simulink model "Model1_Sarah"  (R2023b)
settings: Solver=FixedStepAuto  StartTime=0.0  StopTime=Inf  FixedStep=1e-4  RelTol=1e-3
PostLoadFcn:
  | if any(exist('dsrtsu_mdlpostloadfcn', 'file') ~= 0), dsrtsu_mdlpostloadfcn('Execute', bdroot); end
InitFcn:
  | , if any(exist('rtifpga_mdlclblib', 'file') ~= 0), rtifpga_mdlclblib('Init', bdroot); end,
  | , if any(exist('dsmpb_private', 'file') ~= 0), dsmpb_private('dsmpb_mdlclblib', 'Init', bdroot); end,
  | load('LUT_BRUSA_jax_grad.mat')
  | load('daten_nichtlinear_interpoliert.mat')
  | load('Maschinendaten.mat')
  | load('PI_Controller.mat')
  | load('Nonlinear_IPMSM.mat')
values from neighbouring files (symbols this model uses):
  I_max = 170    [Maschinendaten.mat]    (also in Maschinendaten_Vorgabe.m; test_ModelParameters.m = evalin('base', 'I_max'); test_StrategySelection.m = tc.readConstant(tc.BLK_Imax))
  ID = [-250 -250 -250 -250 -250 -250 -250 -250 -250 -250 -250 -250 ... (10000 elements, 100x100)]    [daten_nichtlinear_interpoliert.mat]
  id_fine = linspace(min(id_vec), max(id_vec), 100)    [Messdaten_Interpoliert.m]    (also in daten_nichtlinear_interpoliert.mat = [-250 -247.474747475 -244.949494949 -242.424242424 -239.8989)
  IQ = [-250 -244.949494949 -239.898989899 -234.848484848 -229.797979798 -224.747474747 -219.696969697 -214.646464646 -209.595959596 -204.545454545 -199.494949495 -194.444444444 ... (10000 elements, 100x100)]    [daten_nichtlinear_interpoliert.mat]
  iq_fine = linspace(min(iq_vec), max(iq_vec), 100)    [Messdaten_Interpoliert.m]    (also in daten_nichtlinear_interpoliert.mat = [-250 -244.949494949 -239.898989899 -234.848484848 -229.7979)
  Ld = Ldd_fine    [Messdaten_Interpoliert.m]    (also in daten_nichtlinear_interpoliert.mat = [0.000225276031415 0.000225750625371 0.000226241749969 0.000)
  Lm = Lm_fine1    [Messdaten_Interpoliert.m]    (also in daten_nichtlinear_interpoliert.mat = [1.34827571578e-05 1.31035668506e-05 1.23153687442e-05 1.146)
  Lq = Lqq_fine    [Messdaten_Interpoliert.m]    (also in daten_nichtlinear_interpoliert.mat = [0.000286039721686 0.000286453471045 0.000286025480511 0.000)
  n_max = 11000    [Maschinendaten.mat]    (also in Maschinendaten_Vorgabe.m; test_ModelParameters.m = evalin('base', 'n_max'); test_StrategySelection.m = tc.readConstant(tc.BLK_nmax))
  p = 3    [Maschinendaten.mat]    (also in Maschinendaten_Vorgabe.m; Messdaten_Interpoliert.m; test_ModelParameters.m = evalin('base', 'p'))
  PSID = Psid_fine    [Messdaten_Interpoliert.m]    (also in daten_nichtlinear_interpoliert.mat = [0.00602681114795 0.00609490588107 0.00615917040906 0.006219)
  PSIQ = PSIQ1 - PSIQ1(iq0_idx,:)    [Messdaten_Interpoliert.m]    (also in daten_nichtlinear_interpoliert.mat = [-0.151946994742 -0.150499709177 -0.149057806808 -0.14762041)
  Rs = 0.018    [Maschinendaten.mat]    (also in Maschinendaten_Vorgabe.m; test_ModelParameters.m = evalin('base', 'Rs'))
  U_dc = 560    [Maschinendaten.mat]    (also in Maschinendaten_Vorgabe.m; test_ModelParameters.m = evalin('base', 'U_dc'))
  U_max = 323.316150746    [Maschinendaten.mat]    (also in Maschinendaten_Vorgabe.m = U_dc / sqrt(3); test_ModelParameters.m = evalin('base', 'U_max'))
libraries: dsmpblib x6
(part 1 of 2)
PreSaveFcn:
  | , if any(exist('dsmpb_private', 'file') ~= 0), dsmpb_private('dsmpb_mdlclblib', 'PreSave', bdroot); end,
CloseFcn:
  | , if any(exist('dsmpb_private', 'file') ~= 0), dsmpb_private('dsmpb_mdlclblib', 'Close', bdroot); end,
settings Model: DSRTSU_INTERNAL_RTIFPGA=210  DSRTSU_INTERNAL_RTISTBM_VER=24.2  DSMPB_ID_DATA={'227',struct('BlockId','b1d00881-2476-43fd-8fde-9f6f39539870396','SignalIds',{{'b1d00881-2476-43fd-8fde-9f6f39539870396_1'}}),'228',struct('BlockId','b1d00881-2476-43fd-8fde-9f6f39539870397','SignalIds',{{'b1d00881-2476-43fd-8fde-9f6f39539870397_1'}}),'229',struct('BlockId','b1d00881-2476-43fd-8fde-9f6f39539870398','SignalIds',{{'b1d00881-2476-43fd-8fde-9f6f39539870398_1'}}),'230',struct('BlockId','b1d00881-2476-43fd-8fde-9f6f39539870399','SignalIds',{{'b1d00881-2476-43fd-8fde-9f6f39539870399_1'}}),'231',struct('BlockId','b1d00881-2476-43fd-8fde-9f6f39539870400','SignalIds',{{'b1d00881-2476-43fd-8fde-9f6f39539870400_1'}}),'232',struct('BlockId','b1d00881-2476-43fd-8fde-9f6f39539870401','SignalIds',{{'b1d00881-2476-43fd-8fde-9f6f39539870401_1'}})}  Creator=Student  LastModifiedBy=Student
settings OptimizationCC: BlockReduction=off  ConditionallyExecuteInputs=off  OptimizeBlockIOStorage=off  BufferReuse=off
settings DebuggingCC: TasksWithSamePriorityMsg=none
settings HardwareCC: ProdBitPerLong=64  ProdLargestAtomicInteger=Integer  ProdWordSize=32  ProdLongLongMode=on  ProdHWDeviceType=Custom Processor->Custom
settings ModelReferenceCC: EnableParallelModelReferenceBuilds=on
settings RTWCC: Description=dSPACE Target DSRT - Generates SIC files for import by ConfigurationDesk and VEOS. Provides code generation for Simulink models imported in ConfigurationDesk.  SystemTargetFile=dsrt.tlc  GenCodeOnly=on  MakeCommand=make_dsrt  TemplateMakefile=dsrt_default_tmf  RTWVerbose=off
settings STFCustomTargetCC: ParMdlRefBuildCompliant=on  SystemTargetFile=dsrt.tlc
settings GRTTargetCC: CompOptLevelCompliant=off  ConcurrentExecutionCompliant=off  CombineOutputUpdateFcns=off  MatFileLogging=off  CPPClassGenCompliant=off  UseToolchainInfoCompliant=off

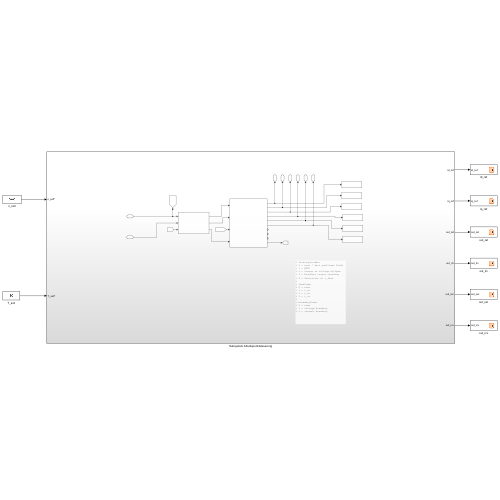
[thumbnail: Simulink's stored preview of the top-level diagram]
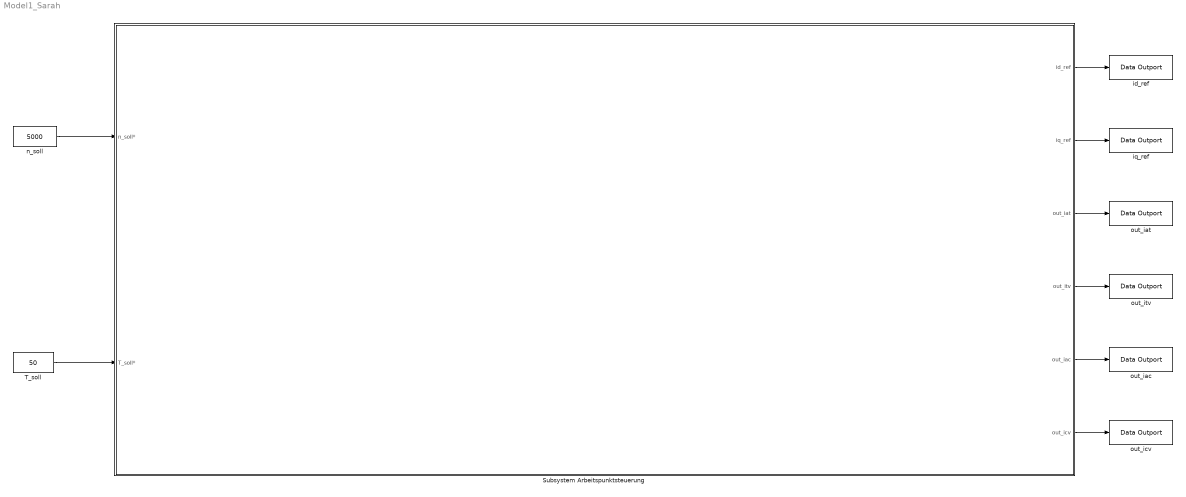
== system Model1_Sarah ==
  Subsystem Arbeitspunktsteuerung : Subsystem
  T_soll : Constant  Value=50
  id_ref : dsmpblib/Data Outport  Priority=-10000
      settings: SourceProductName=dSPACE Model Interface Package for Simulink (MIPS)
  iq_ref : dsmpblib/Data Outport  Priority=-10000
      settings: SourceProductName=dSPACE Model Interface Package for Simulink (MIPS)
  n_soll : Constant  Value=5000
  out_iac : dsmpblib/Data Outport  Priority=-10000
      settings: SourceProductName=dSPACE Model Interface Package for Simulink (MIPS)
  out_iat : dsmpblib/Data Outport  Priority=-10000
      settings: SourceProductName=dSPACE Model Interface Package for Simulink (MIPS)
  out_icv : dsmpblib/Data Outport  Priority=-10000
      settings: SourceProductName=dSPACE Model Interface Package for Simulink (MIPS)
  out_itv : dsmpblib/Data Outport  Priority=-10000
      settings: SourceProductName=dSPACE Model Interface Package for Simulink (MIPS)
  wires:
  Subsystem Arbeitspunktsteuerung/3(out_iat) -> out_iat/1
  Subsystem Arbeitspunktsteuerung/4(out_itv) -> out_itv/1
  Subsystem Arbeitspunktsteuerung/5(out_iac) -> out_iac/1
  Subsystem Arbeitspunktsteuerung/6(out_icv) -> out_icv/1
  n_soll/1 -> Subsystem Arbeitspunktsteuerung/1(n_soll*)
  T_soll/1 -> Subsystem Arbeitspunktsteuerung/2(T_soll*)
  Subsystem Arbeitspunktsteuerung/1(id_ref) -> id_ref/1
  Subsystem Arbeitspunktsteuerung/2(iq_ref) -> iq_ref/1

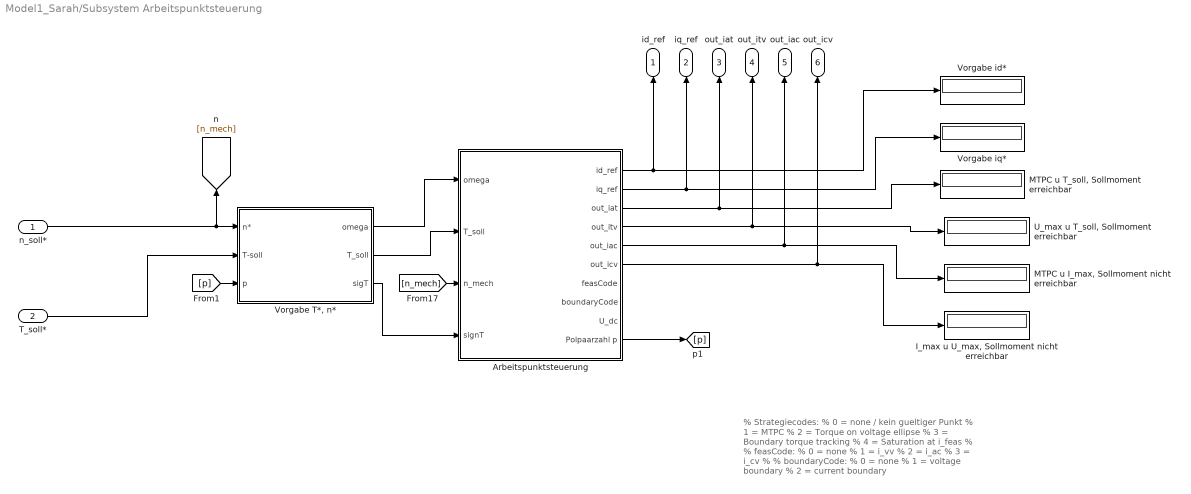
== system Model1_Sarah/Subsystem Arbeitspunktsteuerung ==
  note: % Strategiecodes:
      | % 0 = none / kein gueltiger Punkt
      | % 1 = MTPC
      | % 2 = Torque on voltage ellipse
      | % 3 = Boundary torque tracking
      | % 4 = Saturation at i_feas
      | %
      | % feasCode:
      | % 0 = none
      | % 1 = i_vv
      | % 2 = i_ac
      | % 3 = i_cv
      | %
      | % boundaryCode:
      | % 0 = none
      | % 1 = voltage boundary
      | % 2 = current boundary
  n_soll* : Inport
  T_soll* : Inport  Port=2
  Arbeitspunktsteuerung : Subsystem
  "I_max u U_max, Sollmoment nicht erreichbar" : Display
  "MTPC u I_max, Sollmoment nicht erreichbar" : Display
  "MTPC u T_soll, Sollmoment erreichbar" : Display
  "U_max u T_soll, Sollmoment erreichbar" : Display
  "Vorgabe T*, n*" : Subsystem
  Vorgabe id* : Display
  Vorgabe iq* : Display
  id_ref : Outport
  iq_ref : Outport  Port=2
  out_iat : Outport  Port=3
  out_itv : Outport  Port=4
  out_iac : Outport  Port=5
  out_icv : Outport  Port=6
  wires:
  Arbeitspunktsteuerung/10(Polpaarzahl p) -> [p]
  "Vorgabe T*, n*"/1(omega) -> Arbeitspunktsteuerung/1(omega)
  Arbeitspunktsteuerung/5(out_iac) -> "MTPC u I_max, Sollmoment nicht erreichbar"/1, out_iac/1
  "Vorgabe T*, n*"/3(sigT) -> Arbeitspunktsteuerung/4(signT)
  [n_mech] -> Arbeitspunktsteuerung/3(n_mech)
  Arbeitspunktsteuerung/2(iq_ref) -> Vorgabe iq*/1, iq_ref/1
  Arbeitspunktsteuerung/3(out_iat) -> "MTPC u T_soll, Sollmoment erreichbar"/1, out_iat/1
  Arbeitspunktsteuerung/1(id_ref) -> Vorgabe id*/1, id_ref/1
  Arbeitspunktsteuerung/4(out_itv) -> "U_max u T_soll, Sollmoment erreichbar"/1, out_itv/1
  T_soll*/1 -> "Vorgabe T*, n*"/2(T-soll)
  [p] -> "Vorgabe T*, n*"/3(p)
  "Vorgabe T*, n*"/2(T_soll) -> Arbeitspunktsteuerung/2(T_soll)
  n_soll*/1 -> "Vorgabe T*, n*"/1(n*), [n_mech]
  Arbeitspunktsteuerung/6(out_icv) -> "I_max u U_max, Sollmoment nicht erreichbar"/1, out_icv/1

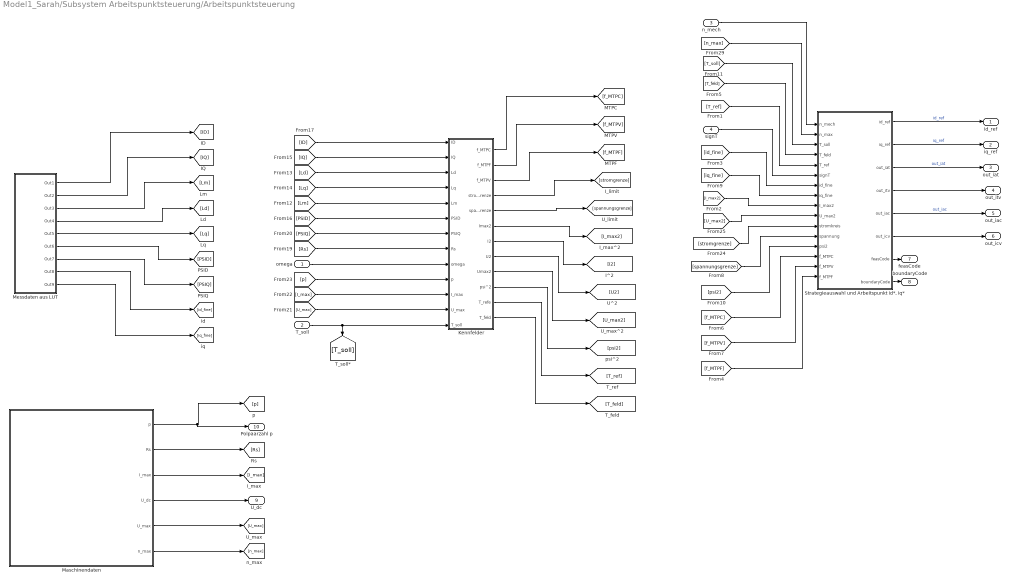
== system Model1_Sarah/Subsystem Arbeitspunktsteuerung/Arbeitspunktsteuerung ==
  omega : Inport
  T_soll : Inport  Port=2
  n_mech : Inport  Port=3
  signT : Inport  Port=4
  Kennfelder : Subsystem  Tag=<DSModel=3_'Model_Sarah'>
      settings: AttributesFormatString=<DSModel='Model_Sarah'>
  Maschinendaten : Subsystem  Tag=<DSModel=5_'Model_Sarah'>
      settings: AttributesFormatString=<DSModel='Model_Sarah'>
  Messdaten aus LUT : Subsystem  Tag=<DSModel=4_'Model_Sarah'>
      settings: AttributesFormatString=<DSModel='Model_Sarah'>
  "Strategieauswahl und Arbeitspunkt id*, iq*" : MATLAB Function  Tag=<DSModel=1_'Model_Sarah'>  TreatAsAtomicUnit=on
      settings: AttributesFormatString=<DSModel='Model_Sarah'>
  id_ref : Outport
  iq_ref : Outport  Port=2
  out_iat : Outport  Port=3
  out_itv : Outport  Port=4
  out_iac : Outport  Port=5
  out_icv : Outport  Port=6
  feasCode : Outport  Port=7
  boundaryCode : Outport  Port=8
  " U_dc" : Outport  Port=9
  Polpaarzahl p : Outport  Port=10
  wires:
  [T_soll] -> "Strategieauswahl und Arbeitspunkt id*, iq*"/3(T_soll)
  "Strategieauswahl und Arbeitspunkt id*, iq*"/7(feasCode) -> feasCode/1
  Kennfelder/9(Umax2) -> [U_max2]
  [stromgrenze] -> "Strategieauswahl und Arbeitspunkt id*, iq*"/11(stromkreis)
  Kennfelder/2(f_MTPF) -> [f_MTPV]
  Messdaten aus LUT/6(Out6) -> [PSID]
  [U_max] -> Kennfelder/12(U_max)
  "Strategieauswahl und Arbeitspunkt id*, iq*"/6(out_icv) -> out_icv/1
  [spannungsgrenze] -> "Strategieauswahl und Arbeitspunkt id*, iq*"/12(spannung)
  Messdaten aus LUT/7(Out7) -> [PSIQ]
  [id_fine] -> "Strategieauswahl und Arbeitspunkt id*, iq*"/7(id_fine)
  Messdaten aus LUT/1(Out1) -> [ID]
  "Strategieauswahl und Arbeitspunkt id*, iq*"/3(out_iat) -> out_iat/1  "out_iat"
  [f_MTPF] -> "Strategieauswahl und Arbeitspunkt id*, iq*"/16(f_MTPF)
  Kennfelder/6(Imax2) -> [I_max2]
  [I_max2] -> "Strategieauswahl und Arbeitspunkt id*, iq*"/9(I_max2)
  signT/1 -> "Strategieauswahl und Arbeitspunkt id*, iq*"/6(signT)
  Messdaten aus LUT/9(Out9) -> [iq_fine]
  "Strategieauswahl und Arbeitspunkt id*, iq*"/5(out_iac) -> out_iac/1  "out_iac"
  omega/1 -> Kennfelder/9(omega)
  Messdaten aus LUT/2(Out2) -> [IQ]
  Maschinendaten/5(U_max) -> [U_max]
  [iq_fine] -> "Strategieauswahl und Arbeitspunkt id*, iq*"/8(iq_fine)
  Kennfelder/8(U2) -> [U2]
  [Lq] -> Kennfelder/4(Lq)
  Kennfelder/3(f_MTPV) -> [f_MTPF]
  [p] -> Kennfelder/10(p)
  Kennfelder/1(f_MTPC) -> [f_MTPC]
  [T_ref] -> "Strategieauswahl und Arbeitspunkt id*, iq*"/5(T_ref)
  "Strategieauswahl und Arbeitspunkt id*, iq*"/2(iq_ref) -> iq_ref/1  "iq_ref"
  Kennfelder/4(stromgrenze) -> [stromgrenze]
  Messdaten aus LUT/8(Out8) -> [id_fine]
  [ID] -> Kennfelder/1(ID)
  Messdaten aus LUT/4(Out4) -> [Ld]
  Kennfelder/12(T_feld) -> [T_feld]
  [psi2] -> "Strategieauswahl und Arbeitspunkt id*, iq*"/13(psi2)
  "Strategieauswahl und Arbeitspunkt id*, iq*"/8(boundaryCode) -> boundaryCode/1
  [PSIQ] -> Kennfelder/7(PSIQ)
  Maschinendaten/1(" p") -> [p], Polpaarzahl p/1
  Maschinendaten/3(" I_max") -> [I_max]
  "Strategieauswahl und Arbeitspunkt id*, iq*"/1(id_ref) -> id_ref/1  "id_ref"
  [f_MTPV] -> "Strategieauswahl und Arbeitspunkt id*, iq*"/15(f_MTPV)
  Kennfelder/5(spannungsgrenze) -> [spannungsgrenze]
  [PSID] -> Kennfelder/6(PSID)
  T_soll/1 -> [T_soll], Kennfelder/13(T_soll)
  [n_max] -> "Strategieauswahl und Arbeitspunkt id*, iq*"/2(n_max)
  Messdaten aus LUT/3(Out3) -> [Lm]
  Kennfelder/11(T_refe) -> [T_ref]
  Messdaten aus LUT/5(Out5) -> [Lq]
  Kennfelder/10(psi^2) -> [psi2]
  [IQ] -> Kennfelder/2(IQ)
  n_mech/1 -> "Strategieauswahl und Arbeitspunkt id*, iq*"/1(n_mech)
  [f_MTPC] -> "Strategieauswahl und Arbeitspunkt id*, iq*"/14(f_MTPC)
  Maschinendaten/6(n_max) -> [n_max]
  [I_max] -> Kennfelder/11(I_max)
  [Lm] -> Kennfelder/5(Lm)
  [T_feld] -> "Strategieauswahl und Arbeitspunkt id*, iq*"/4(T_feld)
  Kennfelder/7(I2) -> [I2]
  Maschinendaten/2(" Rs") -> [Rs]
  Maschinendaten/4(" U_dc") -> " U_dc"/1
  "Strategieauswahl und Arbeitspunkt id*, iq*"/4(out_itv) -> out_itv/1
  [Rs] -> Kennfelder/8(Rs)
  [Ld] -> Kennfelder/3(Ld)
  [U_max2] -> "Strategieauswahl und Arbeitspunkt id*, iq*"/10(U_max2)

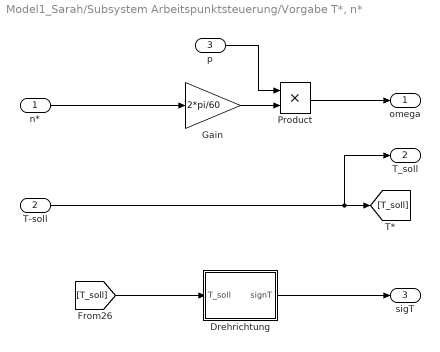
== system Model1_Sarah/Subsystem Arbeitspunktsteuerung/Vorgabe T*, n* ==
  n* : Inport
  T-soll : Inport  Port=2
  p : Inport  Port=3
  Drehrichtung : MATLAB Function  Tag=<DSModel=2_'Model_Sarah'>  TreatAsAtomicUnit=on
      settings: AttributesFormatString=<DSModel='Model_Sarah'>
  Gain : Gain  Gain=2*pi/60
  Product : Product
  omega : Outport
  T_soll : Outport  Port=2
  sigT : Outport  Port=3
  wires:
  p/1 -> Product/1
  Drehrichtung/1(signT) -> sigT/1
  Gain/1 -> Product/2
  n*/1 -> Gain/1
  T-soll/1 -> [T_soll], T_soll/1
  Product/1 -> omega/1
  [T_soll] -> Drehrichtung/1(T_soll)

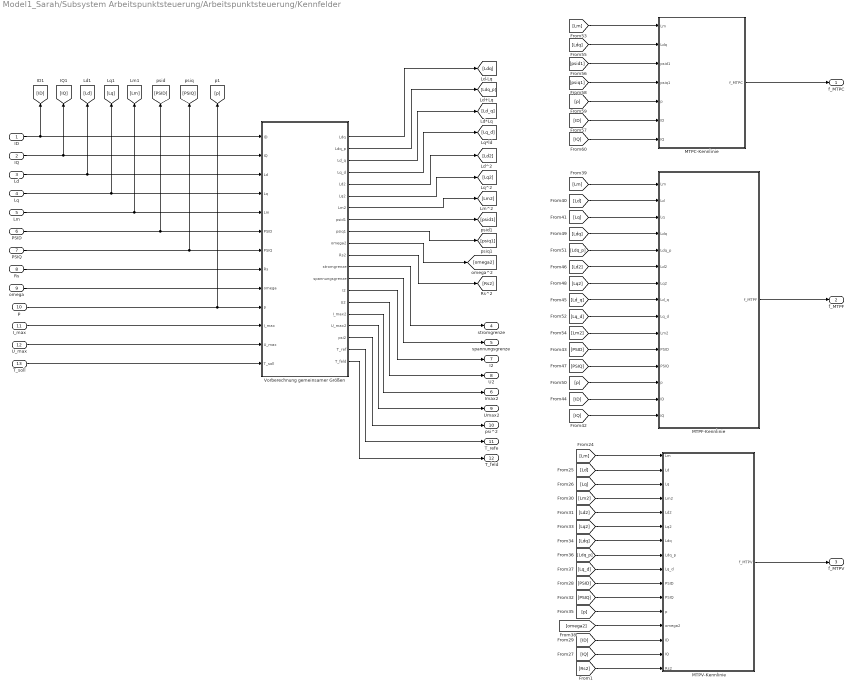
== system Model1_Sarah/Subsystem Arbeitspunktsteuerung/Arbeitspunktsteuerung/Kennfelder ==
  ID : Inport
  IQ : Inport  Port=2
  Ld : Inport  Port=3
  Lq : Inport  Port=4
  Lm : Inport  Port=5
  PSID : Inport  Port=6
  PSIQ : Inport  Port=7
  Rs : Inport  Port=8
  omega : Inport  Port=9
  p : Inport  Port=10
  I_max : Inport  Port=11
  U_max : Inport  Port=12
  T_soll : Inport  Port=13
  " Vorberechnung gemeinsamer Größen" : MATLAB Function  TreatAsAtomicUnit=on
  MTPC-Kennlinie : MATLAB Function  TreatAsAtomicUnit=on
  MTPF-Kennlinie : MATLAB Function  TreatAsAtomicUnit=on
  MTPV-Kennlinie : MATLAB Function  TreatAsAtomicUnit=on
  f_MTPC : Outport
  f_MTPF : Outport  Port=2
  f_MTPV : Outport  Port=3
  stromgrenze : Outport  Port=4
  spannungsgrenze : Outport  Port=5
  Imax2 : Outport  Port=6
  I2 : Outport  Port=7
  U2 : Outport  Port=8
  Umax2 : Outport  Port=9
  psi^2 : Outport  Port=10
  T_refe : Outport  Port=11
  T_feld : Outport  Port=12
  wires:
  T_soll/1 -> " Vorberechnung gemeinsamer Größen"/13(T_soll)
  " Vorberechnung gemeinsamer Größen"/20(T_feld) -> T_feld/1
  " Vorberechnung gemeinsamer Größen"/19(T_ref) -> T_refe/1
  " Vorberechnung gemeinsamer Größen"/18(psi2) -> psi^2/1
  " Vorberechnung gemeinsamer Größen"/16(I_max2) -> Imax2/1
  " Vorberechnung gemeinsamer Größen"/14(I2) -> I2/1
  " Vorberechnung gemeinsamer Größen"/17(U_max2) -> Umax2/1
  " Vorberechnung gemeinsamer Größen"/15(U2) -> U2/1
  [Rs2] -> MTPV-Kennlinie/16(Rs2)
  MTPV-Kennlinie/1(f_MTPV) -> f_MTPV/1
  MTPC-Kennlinie/1(f_MTPC) -> f_MTPC/1
  MTPF-Kennlinie/1(f_MTPF) -> f_MTPF/1
  PSID/1 -> " Vorberechnung gemeinsamer Größen"/6(PSID), [PSID]
  Lm/1 -> " Vorberechnung gemeinsamer Größen"/5(Lm), [Lm]
  U_max/1 -> " Vorberechnung gemeinsamer Größen"/12(U_max)
  Lq/1 -> " Vorberechnung gemeinsamer Größen"/4(Lq), [Lq]
  I_max/1 -> " Vorberechnung gemeinsamer Größen"/11(I_max)
  IQ/1 -> " Vorberechnung gemeinsamer Größen"/2(IQ), [IQ]
  p/1 -> " Vorberechnung gemeinsamer Größen"/10(p), [p]
  PSIQ/1 -> " Vorberechnung gemeinsamer Größen"/7(PSIQ), [PSIQ]
  [Ldq] -> MTPF-Kennlinie/4(Ldq)
  [omega2] -> MTPV-Kennlinie/13(omega2)
  omega/1 -> " Vorberechnung gemeinsamer Größen"/9(omega)
  [Ld2] -> MTPF-Kennlinie/6(Ld2)
  [Lq] -> MTPV-Kennlinie/3(Lq)
  [Lm] -> MTPV-Kennlinie/1(Lm)
  " Vorberechnung gemeinsamer Größen"/7(Lm2) -> [Lm2]
  [Ld] -> MTPF-Kennlinie/2(Ld)
  [Ldq_p] -> MTPV-Kennlinie/8(Ldq_p)
  [Ldq] -> MTPV-Kennlinie/7(Ldq)
  " Vorberechnung gemeinsamer Größen"/3(Ld_q) -> [Ld_q]
  [Lq2] -> MTPV-Kennlinie/6(Lq2)
  [ID] -> MTPV-Kennlinie/14(ID)
  [PSIQ] -> MTPF-Kennlinie/12(PSIQ)
  " Vorberechnung gemeinsamer Größen"/4(Lq_d) -> [Lq_d]
  [p] -> MTPC-Kennlinie/5(p)
  " Vorberechnung gemeinsamer Größen"/8(psid1) -> [psid1]
  [Lq_d] -> MTPV-Kennlinie/9(Lq_d)
  Ld/1 -> " Vorberechnung gemeinsamer Größen"/3(Ld), [Ld]
  [ID] -> MTPF-Kennlinie/14(ID)
  Rs/1 -> " Vorberechnung gemeinsamer Größen"/8(Rs)
  " Vorberechnung gemeinsamer Größen"/1(Ldq) -> [Ldq]
  [Ldq_p] -> MTPF-Kennlinie/5(Ldq_p)
  [IQ] -> MTPV-Kennlinie/15(IQ)
  [PSID] -> MTPV-Kennlinie/10(PSID)
  " Vorberechnung gemeinsamer Größen"/10(omega2) -> [omega2]
  " Vorberechnung gemeinsamer Größen"/13(spannungsgrenze) -> spannungsgrenze/1
  [Lm] -> MTPC-Kennlinie/1(Lm)
  [psiq1] -> MTPC-Kennlinie/4(psiq1)
  [psid1] -> MTPC-Kennlinie/3(psid1)
  [p] -> MTPF-Kennlinie/13(p)
  ID/1 -> " Vorberechnung gemeinsamer Größen"/1(ID), [ID]
  [IQ] -> MTPC-Kennlinie/7(IQ)
  [ID] -> MTPC-Kennlinie/6(ID)
  [IQ] -> MTPF-Kennlinie/15(IQ)
  [Lq2] -> MTPF-Kennlinie/7(Lq2)
  " Vorberechnung gemeinsamer Größen"/12(stromgrenze) -> stromgrenze/1
  " Vorberechnung gemeinsamer Größen"/5(Ld2) -> [Ld2]
  [Ld_q] -> MTPF-Kennlinie/8(Ld_q)
  [Lm] -> MTPF-Kennlinie/1(Lm)
  [PSID] -> MTPF-Kennlinie/11(PSID)
  " Vorberechnung gemeinsamer Größen"/11(Rs2) -> [Rs2]
  [Ld] -> MTPV-Kennlinie/2(Ld)
  " Vorberechnung gemeinsamer Größen"/6(Lq2) -> [Lq2]
  [Lq] -> MTPF-Kennlinie/3(Lq)
  [Lm2] -> MTPF-Kennlinie/10(Lm2)
  [Lq_d] -> MTPF-Kennlinie/9(Lq_d)
  [Ld2] -> MTPV-Kennlinie/5(Ld2)
  [p] -> MTPV-Kennlinie/12(p)
  " Vorberechnung gemeinsamer Größen"/9(psiq1) -> [psiq1]
  [Lm2] -> MTPV-Kennlinie/4(Lm2)
  [PSIQ] -> MTPV-Kennlinie/11(PSIQ)
  " Vorberechnung gemeinsamer Größen"/2(Ldq_p) -> [Ldq_p]
  [Ldq] -> MTPC-Kennlinie/2(Ldq)

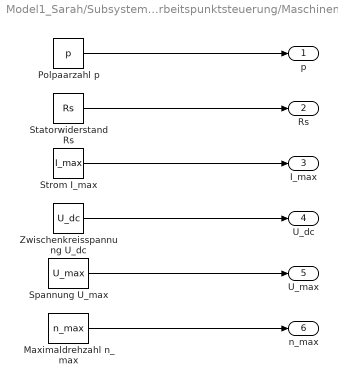
== system Model1_Sarah/Subsystem Arbeitspunktsteuerung/Arbeitspunktsteuerung/Maschinendaten ==
  Maximaldrehzahl n_max : Constant  Value=n_max
  Polpaarzahl p : Constant  Value=p
  Spannung U_max : Constant  Value=U_max
  Statorwiderstand Rs : Constant  Value=Rs
  Strom I_max : Constant  Value=I_max
  Zwischenkreisspannung U_dc : Constant  Value=U_dc
  " p" : Outport
  " Rs" : Outport  Port=2
  " I_max" : Outport  Port=3
  " U_dc" : Outport  Port=4
  U_max : Outport  Port=5
  n_max : Outport  Port=6
  wires:
  Maximaldrehzahl n_max/1 -> n_max/1
  Spannung U_max/1 -> U_max/1
  Statorwiderstand Rs/1 -> " Rs"/1
  Polpaarzahl p/1 -> " p"/1
  Strom I_max/1 -> " I_max"/1
  Zwischenkreisspannung U_dc/1 -> " U_dc"/1

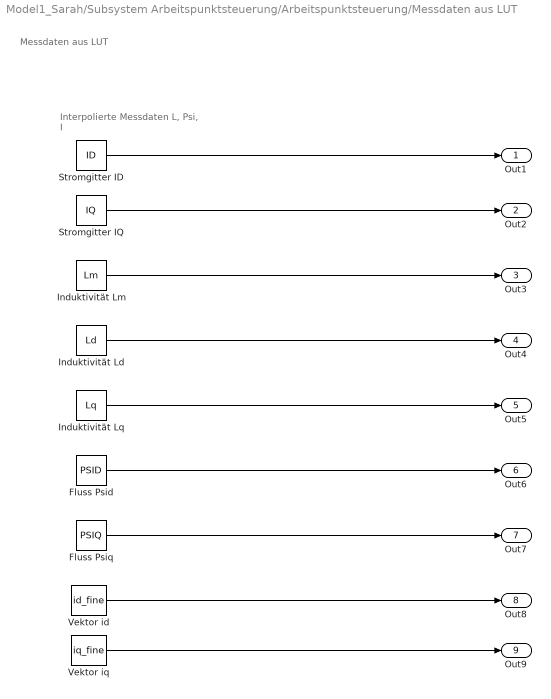
== system Model1_Sarah/Subsystem Arbeitspunktsteuerung/Arbeitspunktsteuerung/Messdaten aus LUT ==
  note: Messdaten aus LUT
  note: Interpolierte Messdaten L, Psi, I
  Fluss Psid : Constant  Value=PSID
  Fluss Psiq : Constant  Value=PSIQ
  Induktivität Ld : Constant  Value=Ld
  Induktivität Lm : Constant  Value=Lm
  Induktivität Lq : Constant  Value=Lq
  Stromgitter ID : Constant  Value=ID
  Stromgitter IQ : Constant  Value=IQ
  Vektor id : Constant  Value=id_fine
  Vektor iq : Constant  Value=iq_fine
  Out1 : Outport
  Out2 : Outport  Port=2
  Out3 : Outport  Port=3
  Out4 : Outport  Port=4
  Out5 : Outport  Port=5
  Out6 : Outport  Port=6
  Out7 : Outport  Port=7
  Out8 : Outport  Port=8
  Out9 : Outport  Port=9
  wires:
  Vektor id/1 -> Out8/1
  Vektor iq/1 -> Out9/1
  Stromgitter ID/1 -> Out1/1
  Stromgitter IQ/1 -> Out2/1
  Fluss Psid/1 -> Out6/1
  Fluss Psiq/1 -> Out7/1
  Induktivität Lm/1 -> Out3/1
  Induktivität Ld/1 -> Out4/1
  Induktivität Lq/1 -> Out5/1

== matlab function Model1_Sarah/Subsystem Arbeitspunktsteuerung/Arbeitspunktsteuerung/Strategieauswahl und Arbeitspunkt id*, iq* ==
  data: n_mech input; n_max input; T_soll input; T_feld input; T_ref input; signT input; id_fine input; iq_fine input; I_max2 input; U_max2 input; stromkreis input; spannung input; psi2 input; f_MTPC input; f_MTPV input; f_MTPF input; id_ref output; iq_ref output; out_iat output; out_itv output; out_iac output; out_icv output; feasCode output; boundaryCode output
%% Strategieauswahl gemäß Flowchart und Bestimmung Arbeitspunkt id*, iq*
% Interpolation, Charak. Punkte, Flowchart-Logik, Nachverfeinerung

%% FUNKTIONIERT NICHT KORREKT STAND 25.06.2026
% Bei T*= 70, n*=10000 wird nicht itv gewählt

function [id_ref, iq_ref, out_iat, out_itv, out_iac, out_icv, feasCode, boundaryCode] = fcn( ...
     n_mech, n_max, T_soll, T_feld, T_ref, signT,...
     id_fine, iq_fine, I_max2, U_max2, ...
     stromkreis,spannung, psi2, f_MTPC, f_MTPV, f_MTPF)

% Strategiecodes, da keine Textausgabe möglich:
% Fälle:
%   out_iat = 1  -> MTPC ∩ T_soll, Sollmoment erreichbar
%   out_itv = 1  -> U_max ∩ T_soll, Sollmoment erreichbar
%   out_iac = 1  -> MTPC ∩ I_max, Sollmoment nicht erreichbar
%   out_icv = 1  -> I_max ∩ U_max, Sollmoment nicht erreichbar
%
% feasCode:
% 0 = none
% 1 = i_vv
% 2 = i_ac
% 3 = i_cv
%
% boundaryCode:
% 0 = none
% 1 = voltage boundary
% 2 = current boundary

%% Konstanten fuer Root-/Mode-Codes
ROOT_AC = 1;
ROOT_VV = 2;
ROOT_AV = 3;
ROOT_CV = 4;
ROOT_AT = 5;
ROOT_TV = 6;

MODE_INTERIOR = 1;
MODE_BOUNDARY = 2;
MODE_VOLTAGE  = 3;

BND_NONE    = 0;
BND_VOLTAGE = 1;
BND_CURRENT = 2;

%% Initialisierung
id_ref = 0.0;
iq_ref = 0.0;
feasCode = int32(0);
boundaryCode = int32(0);

i_ref  = [NaN NaN];
i_feas = [NaN NaN];

out_iat = 0.0;
out_itv = 0.0;
out_iac = 0.0;
out_icv = 0.0;

%% Schutz
if n_mech > n_max
    id_ref = 0.0;
    iq_ref = 0.0;
    feasCode = int32(0);
    boundaryCode = int32(0);
    return;
end

%% 4) Kontext
ctx.xvec   = id_fine;
ctx.yvec   = iq_fine;
ctx.Ti     = T_feld;
ctx.Teql   = T_ref;
ctx.Ieql   = stromkreis;
ctx.Ueql   = spannung;
ctx.Psi2i  = psi2;
ctx.MTPCi  = f_MTPC;
ctx.MTPVi  = f_MTPV;
ctx.MTPFi  = f_MTPF;
ctx.Tref   = T_soll;
ctx.signT  = signT;
ctx.tolEq  = 1e-6 * max([1, I_max2, U_max2, abs(T_soll)]);
ctx.tolT   = max(0.25, 1e-3*max(1, abs(T_soll)));

%% 5) Charakteristische Punkte im Flowchart
pts_iac = findCurveIntersections(id_fine, iq_fine, f_MTPC,    0.0, stromkreis, 0.0, ctx);
pts_ivv = findCurveIntersections(id_fine, iq_fine, f_MTPV,    0.0, spannung,   0.0, ctx);
pts_iav = findCurveIntersections(id_fine, iq_fine, f_MTPC,    0.0, spannung,   0.0, ctx);
pts_icv = findCurveIntersections(id_fine, iq_fine, stromkreis,0.0, spannung,   0.0, ctx);
pts_iat = findCurveIntersections(id_fine, iq_fine, f_MTPC,    0.0, T_ref,  0.0, ctx);
pts_itv = findCurveIntersections(id_fine, iq_fine, T_ref, 0.0, spannung,   0.0, ctx);

i_ac = chooseCorrectRoot(pts_iac, ROOT_AC, ctx);
i_vv = chooseCorrectRoot(pts_ivv, ROOT_VV, ctx);
i_av = chooseCorrectRoot(pts_iav, ROOT_AV, ctx);
i_cv = chooseCorrectRoot(pts_icv, ROOT_CV, ctx);
i_at = chooseCorrectRoot(pts_iat, ROOT_AT, ctx);
i_tv = chooseCorrectRoot(pts_itv, ROOT_TV, ctx);

%% 6) Flowchart-Logik
% ------------------------------------------------------------
% Fall 1: MTPC ∩ T_soll -> i_at
% Nur wenn Sollmoment auf dem MTPC-Zweig noch erreichbar ist
% ------------------------------------------------------------

if isFinitePoint(i_at)
    I_at = evalGI(ctx.Ieql, i_at, ctx);
    U_at = evalGI(ctx.Ueql, i_at, ctx);

    if (I_at <= 1e-5) && (U_at <= 1e-5)
        i_ref = finalFeasiblePolish(i_at, MODE_INTERIOR, ctx);
        out_iat = 1;    % Sollmoment T* auf MTPC
    end
end

% --- falls MTPC ∩ T_soll nicht direkt zulässig ---
if ~isFinitePoint(i_ref)
    % i_feas bestimmen:
    % Vergleich psi_cv und psi_ac:
    %    - psi_cv > psi_ac  -> i_feas = i_ac
    %    - sonst            -> i_feas = i_cv

    if isFinitePoint(i_vv) && evalGI(ctx.Ieql, i_vv, ctx) <= 1e-5
        i_feas = i_vv;
        feasCode = int32(1); % 1 = i_vv
    else
        psi_ac = inf;
        psi_cv = inf;

        if isFinitePoint(i_ac)
            psi_ac = sqrt(max(evalGI(ctx.Psi2i, i_ac, ctx), 0.0));
        end
        if isFinitePoint(i_cv)
            psi_cv = sqrt(max(evalGI(ctx.Psi2i, i_cv, ctx), 0.0));
        end

        if psi_cv > psi_ac
            i_feas = i_ac;
            feasCode = int32(2); % 2 = i_ac
        else
            i_feas = i_cv;
            feasCode = int32(3); % 3 = i_cv
        end
    end

    m_av  = NaN;
    m_max = NaN;

    if isFinitePoint(i_av)
        m_av = evalGI(ctx.Ti, i_av, ctx);
    end
    if isFinitePoint(i_feas)
        m_max = evalGI(ctx.Ti, i_feas, ctx);
    end

    % ------------------------------------------------------------
    % Fall 2: U_max ∩ T_soll  -> i_tv
    % Sollmoment ist auf der Spannungsgrenze noch erreichbar
    % ------------------------------------------------------------
    if isFinitePoint(i_tv) && isfinite(m_max) && abs(T_soll) <= abs(m_max) + ctx.tolT
        i_ref = finalFeasiblePolish(i_tv, MODE_VOLTAGE, ctx);
        out_itv = 1;    % Sollmoment T* auf Umax 
    end

    % ------------------------------------------------------------
    % Fall 3: MTPC ∩ I_max -> i_ac
    % Sollmoment nicht mehr erreichbar, Umschalten auf Stromgrenze
    % sonst: 
    % Fall 4: I_max ∩ U_max -> i_cv
    % Sollmoment nicht mehr erreichbar, Spannungs- und Stromgrenze aktiv
    % ------------------------------------------------------------
    if ~isFinitePoint(i_ref) && isFinitePoint(i_feas)
        i_ref = i_feas;

        if feasCode == int32(2)
            out_iac = 1;        % KEIN Sollmoment T*, Arbeitspunkt auf MTPC bei Imax
        elseif feasCode == int32(3)
            out_icv = 1;        % KEIN Sollmoment T*,  ARbeitspunkt am Schnittpunkt Imax und Umax
        end
    end
end

%% 7) Schluss-Nachverfeinerung
if isFinitePoint(i_ref)
   if out_itv == 1
       i_ref = refineOnBoundary(i_ref, BND_VOLTAGE, ctx);
  elseif out_iat == 1
       i_ref = finalFeasiblePolish(i_ref, MODE_INTERIOR, ctx);

   elseif out_iac == 1 || out_icv == 1
      % Saettigungs- bzw. Grenzpunkt nicht unnoetig wegziehen
 end
end

%% 8) Ausgaenge
if isFinitePoint(i_ref)
    id_ref = i_ref(1);
    iq_ref = i_ref(2);
else
    id_ref = 0.0;
    iq_ref = 0.0;
end

end

%% == lokale Hilfsfunktionen ===========================================

function z = evalGI(G, p, ctx)
    z = interp2_bilinear_clamped(ctx.xvec, ctx.yvec, G, p(1), p(2));
end

% ========================================================================
function tf = isFinitePoint(p)
    tf = isnumeric(p) && numel(p)==2 && all(isfinite(p));
end

% ========================================================================
function pts = findCurveIntersections(xvec, yvec, F1, lev1, F2, lev2, ctx)

    MAX_PTS = 24;
    pts = nan(MAX_PTS, 2);
    nPts = 0;

    A = F1 - lev1;
    B = F2 - lev2;

    nx = numel(xvec);
    ny = numel(yvec);

    dxMin = min(abs(diff(xvec)));
    dyMin = min(abs(diff(yvec)));
    tolMerge = 0.25 * min(dxMin, dyMin);

    scaleA = max(1.0, max(abs(A(:))));
    scaleB = max(1.0, max(abs(B(:))));
    tolRes = 1e-4;

    for r = 1:ny-1
        for c = 1:nx-1

            Ac = [A(r,c), A(r,c+1), A(r+1,c), A(r+1,c+1)];
            Bc = [B(r,c), B(r,c+1), B(r+1,c), B(r+1,c+1)];

            crossA = (min(Ac) <= 0) && (max(Ac) >= 0);
            crossB = (min(Bc) <= 0) && (max(Bc) >= 0);

            if ~(crossA && crossB)
                continue;
            end

            x0 = 0.5 * (xvec(c) + xvec(c+1));
            y0 = 0.5 * (yvec(r) + yvec(r+1));
            p0 = [x0, y0];

            p1 = localRefine2D(p0, A, B, xvec, yvec, 4, 11);
            p2 = localRefineGN(p1, A, B, xvec, yvec);

            a2 = interp2_bilinear_clamped(xvec, yvec, A, p2(1), p2(2)) / scaleA;
            b2 = interp2_bilinear_clamped(xvec, yvec, B, p2(1), p2(2)) / scaleB;
            res = sqrt(a2*a2 + b2*b2);

            if res < tolRes
                if ~pointExists(pts, p2, tolMerge)
                    nPts = nPts + 1;
                    if nPts <= MAX_PTS
                        pts(nPts,:) = p2;
                    end
                end
            end
        end
    end

    for k = 1:MAX_PTS
        if all(isfinite(pts(k,:)))
            v1 = evalGI(A, pts(k,:), ctx);
            v2 = evalGI(B, pts(k,:), ctx);
            if ~(isfinite(v1) && isfinite(v2))
                pts(k,:) = [NaN NaN];
            end
        end
    end
end

% ========================================================================
function tf = pointExists(pts, p, tol)
    tf = false;
    for k = 1:size(pts,1)
        if all(isfinite(pts(k,:)))
            d = hypot(pts(k,1)-p(1), pts(k,2)-p(2));
            if d <= tol
                tf = true;
                return;
            end
        end
    end
end

% ========================================================================
function xBest = localRefine2D(x0, F1i, F2i, xvec, yvec, nIter, nGrid)

    xBest = x0(:).';

    dx0 = min(abs(diff(xvec)));
    dy0 = min(abs(diff(yvec)));

    hx = 2*dx0;
    hy = 2*dy0;

    s1 = max(1.0, max(abs(F1i(:))));
    s2 = max(1.0, max(abs(F2i(:))));

    for it = 1:nIter
        xL = max(min(xvec), xBest(1)-hx);
        xU = min(max(xvec), xBest(1)+hx);
        yL = max(min(yvec), xBest(2)-hy);
        yU = min(max(yvec), xBest(2)+hy);

        bestE = inf;
        bestX = xBest(1);
        bestY = xBest(2);

        for iy = 0:nGrid-1
            if nGrid == 1
                yq = 0.5*(yL+yU);
            else
                yq = yL + (yU-yL) * (iy/(nGrid-1));
            end

            for ix = 0:nGrid-1
                if nGrid == 1
                    xq = 0.5*(xL+xU);
                else
                    xq = xL + (xU-xL) * (ix/(nGrid-1));
                end

                z1 = interp2_bilinear_clamped(xvec, yvec, F1i, xq, yq) / s1;
                z2 = interp2_bilinear_clamped(xvec, yvec, F2i, xq, yq) / s2;
                E  = z1*z1 + z2*z2;

                if E < bestE
                    bestE = E;
                    bestX = xq;
                    bestY = yq;
                end
            end
        end

        xBest = [bestX, bestY];
        hx = hx/3;
        hy = hy/3;
    end
end

% ========================================================================
function xBest = localRefineGN(x0, F1i, F2i, xvec, yvec)

    x = x0(1);
    y = x0(2);

    lbx = min(xvec); ubx = max(xvec);
    lby = min(yvec); uby = max(yvec);

    dx = min(abs(diff(xvec)));
    dy = min(abs(diff(yvec)));

    sx = max(1e-6, 0.25*dx);
    sy = max(1e-6, 0.25*dy);

    s1 = max(1.0, max(abs(F1i(:))));
    s2 = max(1.0, max(abs(F2i(:))));

    lambda = 1e-6;

    for it = 1:12
        f1 = interp2_bilinear_clamped(xvec, yvec, F1i, x, y) / s1;
        f2 = interp2_bilinear_clamped(xvec, yvec, F2i, x, y) / s2;

        f1xp = interp2_bilinear_clamped(xvec, yvec, F1i, clampScalar(x+sx,lbx,ubx), y) / s1;
        f1xm = interp2_bilinear_clamped(xvec, yvec, F1i, clampScalar(x-sx,lbx,ubx), y) / s1;
        f1yp = interp2_bilinear_clamped(xvec, yvec, F1i, x, clampScalar(y+sy,lby,uby)) / s1;
        f1ym = interp2_bilinear_clamped(xvec, yvec, F1i, x, clampScalar(y-sy,lby,uby)) / s1;

        f2xp = interp2_bilinear_clamped(xvec, yvec, F2i, clampScalar(x+sx,lbx,ubx), y) / s2;
        f2xm = interp2_bilinear_clamped(xvec, yvec, F2i, clampScalar(x-sx,lbx,ubx), y) / s2;
        f2yp = interp2_bilinear_clamped(xvec, yvec, F2i, x, clampScalar(y+sy,lby,uby)) / s2;
        f2ym = interp2_bilinear_clamped(xvec, yvec, F2i, x, clampScalar(y-sy,lby,uby)) / s2;

        j11 = (f1xp - f1xm) / (2*sx);
        j12 = (f1yp - f1ym) / (2*sy);
        j21 = (f2xp - f2xm) / (2*sx);
        j22 = (f2yp - f2ym) / (2*sy);

        h11 = j11*j11 + j21*j21 + lambda;
        h12 = j11*j12 + j21*j22;
        h22 = j12*j12 + j22*j22 + lambda;

        g1 = j11*f1 + j21*f2;
        g2 = j12*f1 + j22*f2;

        detH = h11*h22 - h12*h12;
        if abs(detH) < 1e-16
            break;
        end

        dxStep = -( h22*g1 - h12*g2 ) / detH;
        dyStep = -( -h12*g1 + h11*g2 ) / detH;

        dxStep = clampScalar(dxStep, -dx, dx);
        dyStep = clampScalar(dyStep, -dy, dy);

        xNew = clampScalar(x + dxStep, lbx, ubx);
        yNew = clampScalar(y + dyStep, lby, uby);

        oldObj = f1*f1 + f2*f2;
        nf1 = interp2_bilinear_clamped(xvec, yvec, F1i, xNew, yNew) / s1;
        nf2 = interp2_bilinear_clamped(xvec, yvec, F2i, xNew, yNew) / s2;
        newObj = nf1*nf1 + nf2*nf2;

        if newObj < oldObj
            x = xNew;
            y = yNew;
            lambda = max(1e-10, 0.3*lambda);
        else
            lambda = min(1e2, 10*lambda);
        end

        if hypot(dxStep, dyStep) < 1e-10
            break;
        end
    end

    xBest = [x, y];
end

% ========================================================================
function p = chooseCorrectRoot(points, labelCode, ctx)

    p = [NaN NaN];
    scoreBest = inf;

    for k = 1:size(points,1)
        x = points(k,:);
        if ~all(isfinite(x))
            continue;
        end

        Te = evalGI(ctx.Ti,   x, ctx);
        Ie = evalGI(ctx.Ieql, x, ctx);
        Ue = evalGI(ctx.Ueql, x, ctx);
        ps = sqrt(max(evalGI(ctx.Psi2i, x, ctx),0.0));
        iq = x(2);
        Iabs = hypot(x(1), x(2));

        branchPenalty = 0.0;
        if sign(iq) ~= ctx.signT
            branchPenalty = 100.0;
        end

        feasiblePenalty = 0.0;
        if Ie > 1e-6
            feasiblePenalty = feasiblePenalty + 10.0*Ie;
        end
        if Ue > 1e-6
            feasiblePenalty = feasiblePenalty + 10.0*Ue;
        end

        switch labelCode
            case 1  % ac
                score = abs(Ie) + 0.01*max(Ue,0.0) + branchPenalty + 1e-5*Iabs;
            case 2  % vv
                score = abs(Ue) + 0.01*max(Ie,0.0) + branchPenalty - 1e-6*ctx.signT*Te;
            case 3  % av
                score = abs(Ue) + branchPenalty + 1e-6*Iabs + 0.01*max(Ie,0.0);
            case 4  % cv
                score = abs(Ie) + abs(Ue) + branchPenalty + 1e-6*ps;
            case 5  % at
                score = abs(Te - ctx.Tref) + feasiblePenalty + branchPenalty + 1e-6*Iabs;
            case 6  % tv
                score = abs(Te - ctx.Tref) + abs(Ue) + 0.05*max(Ie,0.0) + branchPenalty;
            otherwise
                score = abs(Te - ctx.Tref) + feasiblePenalty + branchPenalty;
        end

        if score < scoreBest
            scoreBest = score;
            p = x;
        end
    end
end

% ========================================================================
function [pref, boundaryCode] = solveTorqueOnFeasibleBoundary(ctx)

    Vpts = collectBoundaryPoints(ctx.xvec, ctx.yvec, ctx.Ueql, ctx);
    Cpts = collectBoundaryPoints(ctx.xvec, ctx.yvec, ctx.Ieql, ctx);

    MAX_CAND = 512;
    cand = nan(MAX_CAND,2);
    tag  = zeros(MAX_CAND,1);
    nCand = 0;

    for k = 1:size(Vpts,1)
        p = Vpts(k,:);
        if ~all(isfinite(p))
            continue;
        end
        Ie = evalGI(ctx.Ieql, p, ctx);
        T  = evalGI(ctx.Ti,   p, ctx);
        if Ie <= 1e-5 && (sign(T)==ctx.signT || abs(T)<=ctx.tolT)
            nCand = nCand + 1;
            if nCand <= MAX_CAND
                cand(nCand,:) = p;
                tag(nCand) = 1;
            end
        end
    end

    for k = 1:size(Cpts,1)
        p = Cpts(k,:);
        if ~all(isfinite(p))
            continue;
        end
        Ue = evalGI(ctx.Ueql, p, ctx);
        T  = evalGI(ctx.Ti,   p, ctx);
        if Ue <= 1e-5 && (sign(T)==ctx.signT || abs(T)<=ctx.tolT)
            nCand = nCand + 1;
            if nCand <= MAX_CAND
                cand(nCand,:) = p;
                tag(nCand) = 2;
            end
        end
    end

    pref = [NaN NaN];
    boundaryCode = int32(0);

    if nCand == 0
        return;
    end

    bestJ = inf;
    bestIdx = 0;

    for k = 1:nCand
        T = evalGI(ctx.Ti, cand(k,:), ctx);
        J = abs(T - ctx.Tref);
        if J < bestJ
            bestJ = J;
            bestIdx = k;
        end
    end

    p0 = cand(bestIdx,:);

    if tag(bestIdx) == 1
        boundaryCode = int32(1);
        pref = refineOnBoundary(p0, 1, ctx);
    else
        boundaryCode = int32(2);
        pref = refineOnBoundary(p0, 2, ctx);
    end
end

% ========================================================================
function pts = collectBoundaryPoints(xvec, yvec, G, ctx)

    MAX_PTS = 600;
    pts = nan(MAX_PTS,2);
    nPts = 0;

    nx = numel(xvec);
    ny = numel(yvec);
    tolMerge = 0.20*min([min(abs(diff(xvec))), min(abs(diff(yvec)))]);

    for r = 1:ny-1
        for c = 1:nx-1

            x1 = xvec(c);   x2 = xvec(c+1);
            y1 = yvec(r);   y2 = yvec(r+1);

            g11 = G(r,c);
            g12 = G(r,c+1);
            g21 = G(r+1,c);
            g22 = G(r+1,c+1);

            [ok, p] = edgeZeroPoint(x1,y1,g11, x2,y1,g12);
            if ok
                p = localProjectSingleCurve(p, G, xvec, yvec);
                if keepBoundaryPoint(p, pts, tolMerge, ctx)
                    nPts = nPts + 1;
                    if nPts <= MAX_PTS
                        pts(nPts,:) = p;
                    end
                end
            end

            [ok, p] = edgeZeroPoint(x2,y1,g12, x2,y2,g22);
            if ok
                p = localProjectSingleCurve(p, G, xvec, yvec);
                if keepBoundaryPoint(p, pts, tolMerge, ctx)
                    nPts = nPts + 1;
                    if nPts <= MAX_PTS
                        pts(nPts,:) = p;
                    end
                end
            end

            [ok, p] = edgeZeroPoint(x1,y2,g21, x2,y2,g22);
            if ok
                p = localProjectSingleCurve(p, G, xvec, yvec);
                if keepBoundaryPoint(p, pts, tolMerge, ctx)
                    nPts = nPts + 1;
                    if nPts <= MAX_PTS
                        pts(nPts,:) = p;
                    end
                end
            end

            [ok, p] = edgeZeroPoint(x1,y1,g11, x1,y2,g21);
            if ok
                p = localProjectSingleCurve(p, G, xvec, yvec);
                if keepBoundaryPoint(p, pts, tolMerge, ctx)
                    nPts = nPts + 1;
                    if nPts <= MAX_PTS
                        pts(nPts,:) = p;
                    end
                end
            end
        end
    end
end

% ========================================================================
function tf = keepBoundaryPoint(p, pts, tolMerge, ctx)

    tf = false;
    if ~all(isfinite(p))
        return;
    end

    T = evalGI(ctx.Ti, p, ctx);
    if ~((sign(T)==ctx.signT) || (abs(T)<=ctx.tolT))
        return;
    end

    for k = 1:size(pts,1)
        if all(isfinite(pts(k,:)))
            if hypot(pts(k,1)-p(1), pts(k,2)-p(2)) <= tolMerge
                return;
            end
        end
    end

    tf = true;
end

% ========================================================================
function [ok, p] = edgeZeroPoint(x1,y1,g1, x2,y2,g2)

    ok = false;
    p = [NaN NaN];

    if ~isfinite(g1) || ~isfinite(g2)
        return;
    end

    if g1 == 0
        ok = true;
        p = [x1 y1];
        return;
    elseif g2 == 0
        ok = true;
        p = [x2 y2];
        return;
    elseif (g1 < 0 && g2 > 0) || (g1 > 0 && g2 < 0)
        t = g1 / (g1 - g2);
        p = [x1 + t*(x2-x1), y1 + t*(y2-y1)];
        ok = true;
    end
end

% ========================================================================
function p = localProjectSingleCurve(p0, G, xvec, yvec)

    x = p0(1);
    y = p0(2);

    lbx = min(xvec); ubx = max(xvec);
    lby = min(yvec); uby = max(yvec);

    dx = min(abs(diff(xvec)));
    dy = min(abs(diff(yvec)));

    hx = max(1e-6, 0.25*dx);
    hy = max(1e-6, 0.25*dy);

    for it = 1:6
        g  = interp2_bilinear_clamped(xvec, yvec, G, x, y);
        gx = (interp2_bilinear_clamped(xvec, yvec, G, clampScalar(x+hx,lbx,ubx), y) ...
            - interp2_bilinear_clamped(xvec, yvec, G, clampScalar(x-hx,lbx,ubx), y)) / (2*hx);
        gy = (interp2_bilinear_clamped(xvec, yvec, G, x, clampScalar(y+hy,lby,uby)) ...
            - interp2_bilinear_clamped(xvec, yvec, G, x, clampScalar(y-hy,lby,uby))) / (2*hy);

        den = gx*gx + gy*gy;
        if den < 1e-16
            break;
        end

        alpha = g / den;
        x = clampScalar(x - alpha*gx, lbx, ubx);
        y = clampScalar(y - alpha*gy, lby, uby);

        if abs(g) < 1e-10
            break;
        end
    end

    p = [x y];
end

% ========================================================================
function p = refineOnBoundary(p0, btype, ctx)

    p = p0;

    for it = 1:12
        J0 = boundaryObjective(p, btype, ctx, min(ctx.xvec), max(ctx.xvec), min(ctx.yvec), max(ctx.yvec));

        dx = min(abs(diff(ctx.xvec)));
        dy = min(abs(diff(ctx.yvec)));

        cand = [ ...
            p(1)+0.5*dx, p(2);
            p(1)-0.5*dx, p(2);
            p(1), p(2)+0.5*dy;
            p(1), p(2)-0.5*dy;
            p(1)+0.25*dx, p(2)+0.25*dy;
            p(1)+0.25*dx, p(2)-0.25*dy;
            p(1)-0.25*dx, p(2)+0.25*dy;
            p(1)-0.25*dx, p(2)-0.25*dy];

        bestP = p;
        bestJ = J0;

        for k = 1:size(cand,1)
            q = cand(k,:);
            q(1) = clampScalar(q(1), min(ctx.xvec), max(ctx.xvec));
            q(2) = clampScalar(q(2), min(ctx.yvec), max(ctx.yvec));
            Jq = boundaryObjective(q, btype, ctx, min(ctx.xvec), max(ctx.xvec), min(ctx.yvec), max(ctx.yvec));
            if Jq < bestJ
                bestJ = Jq;
                bestP = q;
            end
        end

        if all(abs(bestP - p) < 1e-10)
            break;
        end
        p = bestP;
    end
end

% ========================================================================
function J = boundaryObjective(x, btype, ctx, lbx, ubx, lby, uby)

    xd = clampScalar(x(1), lbx, ubx);
    yq = clampScalar(x(2), lby, uby);
    p  = [xd yq];

    T  = evalGI(ctx.Ti,   p, ctx);
    Ie = evalGI(ctx.Ieql, p, ctx);
    Ue = evalGI(ctx.Ueql, p, ctx);

    Jt = (T - ctx.Tref)^2;

    switch btype
        case 1
            Jb = 1e6*(Ue^2) + 1e7*(max(Ie,0.0)^2);
        case 2
            Jb = 1e6*(Ie^2) + 1e7*(max(Ue,0.0)^2);
        otherwise
            Jb = 1e6*(Ie^2 + Ue^2);
    end

    Jbranch = 0.0;
    if sign(yq) ~= ctx.signT
        Jbranch = 1e5;
    end

    J = Jt + Jb + Jbranch;
end

% ========================================================================
function p = finalFeasiblePolish(p0, mode, ctx)

    p = p0;

    for it = 1:12
        J0 = finalObjective(p, mode, ctx, min(ctx.xvec), max(ctx.xvec), min(ctx.yvec), max(ctx.yvec));

        dx = min(abs(diff(ctx.xvec)));
        dy = min(abs(diff(ctx.yvec)));

        cand = [ ...
            p(1)+0.5*dx, p(2);
            p(1)-0.5*dx, p(2);
            p(1), p(2)+0.5*dy;
            p(1), p(2)-0.5*dy;
            p(1)+0.25*dx, p(2)+0.25*dy;
            p(1)+0.25*dx, p(2)-0.25*dy;
            p(1)-0.25*dx, p(2)+0.25*dy;
            p(1)-0.25*dx, p(2)-0.25*dy];

        bestP = p;
        bestJ = J0;

        for k = 1:size(cand,1)
            q = cand(k,:);
            q(1) = clampScalar(q(1), min(ctx.xvec), max(ctx.xvec));
            q(2) = clampScalar(q(2), min(ctx.yvec), max(ctx.yvec));
            Jq = finalObjective(q, mode, ctx, min(ctx.xvec), max(ctx.xvec), min(ctx.yvec), max(ctx.yvec));
            if Jq < bestJ
                bestJ = Jq;
                bestP = q;
            end
        end

        if all(abs(bestP - p) < 1e-10)
            break;
        end
        p = bestP;
    end
end

% ========================================================================
function J = finalObjective(x, mode, ctx, lbx, ubx, lby, uby)

    xd = clampScalar(x(1), lbx, ubx);
    yq = clampScalar(x(2), lby, uby);
    p  = [xd yq];

    T  = evalGI(ctx.Ti,   p, ctx);
    Ie = evalGI(ctx.Ieql, p, ctx);
    Ue = evalGI(ctx.Ueql, p, ctx);

    Jt = (T - ctx.Tref)^2;
    Jf = 1e7*(max(Ie,0.0)^2 + max(Ue,0.0)^2);

    if sign(yq) ~= ctx.signT
        Jf = Jf + 1e5;
    end

    switch mode
        case 1
            J = Jt + Jf;
        case 2
            J = Jt + 1e6*(min(Ie^2, Ue^2)) + Jf;
        case 3
            J = Jt + 1e6*(Ue^2) + 1e7*(max(Ie,0.0)^2);
        otherwise
            J = Jt + Jf;
    end
end

% ========================================================================
function z = interp2_bilinear_clamped(xvec, yvec, F, x, y)

    nx = numel(xvec);
    ny = numel(yvec);

    x = clampScalar(x, xvec(1), xvec(nx));
    y = clampScalar(y, yvec(1), yvec(ny));

    ix = findInterval(xvec, x);
    iy = findInterval(yvec, y);

    if ix >= nx
        ix = nx - 1;
    end
    if iy >= ny
        iy = ny - 1;
    end

    x1 = xvec(ix);
    x2 = xvec(ix+1);
    y1 = yvec(iy);
    y2 = yvec(iy+1);

    if x2 == x1
        tx = 0.0;
    else
        tx = (x - x1) / (x2 - x1);
    end

    if y2 == y1
        ty = 0.0;
    else
        ty = (y - y1) / (y2 - y1);
    end

    f11 = F(iy,   ix);
    f21 = F(iy,   ix+1);
    f12 = F(iy+1, ix);
    f22 = F(iy+1, ix+1);

    z1 = f11 + tx*(f21 - f11);
    z2 = f12 + tx*(f22 - f12);
    z  = z1 + ty*(z2 - z1);
end

% ========================================================================
function idx = findInterval(vec, x)

    n = numel(vec);

    if x <= vec(1)
        idx = 1;
        return;
    end

    if x >= vec(n)
        idx = n - 1;
        return;
    end

    idx = 1;
    for k = 1:n-1
        if x >= vec(k) && x <= vec(k+1)
            idx = k;
            return;
        end
    end

    idx = n - 1;
end

% ========================================================================
function y = clampScalar(x, lo, hi)
    y = min(max(x, lo), hi);
end
% ========================================================================

== matlab function Model1_Sarah/Subsystem Arbeitspunktsteuerung/Arbeitspunktsteuerung/Kennfelder/ Vorberechnung gemeinsamer Größen ==
  data: ID input; IQ input; Ld input; Lq input; Lm input; PSID input; PSIQ input; Rs input; omega input; p input; I_max input; U_max input; Ldq output; Ldq_p output; Ld_q output; Lq_d output; Ld2 output; Lq2 output; Lm2 output; psid1 output; psiq1 output; omega2 output; Rs2 output; stromgrenze output; spannungsgrenze output; I2 output; U2 output; I_max2 output; U_max2 output; psi2 output; T_ref output; T_feld output; T_soll input
%% 4) Vorberechnung gemeinsamer Größen
% Dieser Block dient der Laufzeitoptimierung.
% Alle häufig benötigten Terme werden einmal zentral berechnet und später
% wiederverwendet. So werden Mehrfachrechnungen vermieden.

function [Ldq, Ldq_p, Ld_q, Lq_d, Ld2, Lq2, Lm2, psid1, psiq1, omega2, Rs2, stromgrenze, spannungsgrenze, I2, U2, I_max2, U_max2, psi2, T_ref, T_feld] = fcn(ID, IQ, Ld, Lq, Lm, PSID, PSIQ, Rs, omega, p, I_max, U_max, T_soll)

% Strom und Spannungsgrenzen
ID2   = ID.^2;
IQ2   = IQ.^2;
IDIQ  = ID.*IQ;

% Maschinenparameter
Ldq = Ld - Lq;      % Differenz Ld - Lq
Ldq_p = Ld + Lq;    % Summe Ld + Lq
Ld_q = Ld.*Lq;      % Matrixmultiplikation Ld.* Lq
Lq_d = Lq.*Ld;      % Matrixmultiplikation Lq.* Ld
Ld2 = Ld.^2;        % Quadrat Ld
Lq2 = Lq.^2;        % Quadrat Lq
Lm2 = Lm.^2;        % Quadrat Lm
psid1 = 1.5*p*PSID; % Vorfaktor PSID
psiq1 = 1.5*p*PSIQ; % Vorfaktor PSIQ
omega2 = omega^2;   % Quadrat Omega
Rs2 = Rs^2;         % Quadrat Rs

% Spannungsanteile in d- und q-Richtung
ud = Rs .* ID - omega .* PSIQ;
uq = Rs .* IQ + omega .* PSID;

% Quadrat von Strom- und Spannungsbetrag
I2 = ID2 + IQ2;
U2 = ud.^2 + uq.^2;

I_max2 = I_max^2;
U_max2 = U_max^2;

% Grenzfunktionen:
stromkreis = I2 - I_max2; % Stromkreis (Betragsgrenze)
spannung   = U2 - U_max2; % Spannungsellipse
stromgrenze = stromkreis;
spannungsgrenze = spannung;

% Flussbetrag
psi2 = PSID.^2 + PSIQ.^2;

% Drehmoment
T_feld = 1.5*p .* ( ...
      PSID.*IQ ...
    - PSIQ.*ID ...
    + (Ld - Lq).*ID.*IQ ...
    + Lm.*(IQ2 - ID2) );

% Referenz-Drehmomenthyperbel
T_ref = T_feld - T_soll;

== matlab function Model1_Sarah/Subsystem Arbeitspunktsteuerung/Arbeitspunktsteuerung/Kennfelder/MTPC-Kennlinie ==
  data: Lm input; f_MTPC output; Ldq input; psid1 input; psiq1 input; p input; ID input; IQ input
%% MTPC Kennlinie 
% konstant, da nur abhängig von Induktivitäten und Flüssen  
function f_MTPC = fcn(Lm, Ldq, psid1, psiq1, p, ID, IQ)

M11 = (Ldq)./2;
M12 = Lm;
M22 = -(Ldq)./2;
mc1 = psid1./4;
mc2 = psiq1./4;

f_MTPC = 1.5*p*(M11.*ID.^2 + 2*M12.*ID.*IQ + M22.*IQ.^2)...
         + 2*(mc1.*ID + mc2.*IQ);

== matlab function Model1_Sarah/Subsystem Arbeitspunktsteuerung/Vorgabe T*, n*/Drehrichtung ==
  data: T_soll input; signT output
%% Vorzeichen Drehmoment -> Festlegung Drehrichtung
function signT = fcn(T_soll)

signT = sign(T_soll);
if signT == 0
    signT = 1;
end

== matlab function Model1_Sarah/Subsystem Arbeitspunktsteuerung/Arbeitspunktsteuerung/Kennfelder/MTPF-Kennlinie ==
  data: Lm input; f_MTPF output; Ld input; Lq input; Ldq input; Ldq_p input; Ld2 input; Lq2 input; Ld_q input; Lq_d input; Lm2 input; PSID input; PSIQ input; p input; ID input; IQ input
%% MTPF Kennlinie 
% konstant, da nur abhängig von Induktivitäten und Flüssen
function f_MTPF = fcn(Lm, Ld, Lq, Ldq, Ldq_p, Ld2, Lq2, Ld_q, Lq_d, Lm2, PSID, PSIQ, p, ID, IQ)

Mf11 = (Ldq)./2 .*(Ld2 + Lm2) + Lm2 .*(Ldq_p);
Mf12 = Lm./2.*(Ld2 + Lq2 + 2*Lm2);
Mf22 = -(Ldq)./2 .*(Lq2 + Lm2) + Lm2 .*(Ldq_p);

mf1 = 1.5*p*((2*Ld2 - Lq_d + 3*Lm2).*PSID./4 ...
      + Lm.* (Ldq_p).*PSIQ./2);
mf2 = 1.5*p*(Lm.* (Ldq_p).*PSID./2 ...
      + (2*Lq2 - Ld_q + 3*Lm2).*PSIQ./4);

my_f = 0.75*p*(Ld.*(PSID).^2 + 2*Lm.*PSID.*PSIQ + Lq.*(PSIQ).^2);

f_MTPF = 1.5*p*(Mf11.*ID.^2 + 2*Mf12.*ID.*IQ + Mf22.*IQ.^2)...
         + 2*(mf1.*ID + mf2.*IQ) + my_f;
